simulink model "DCmotor_single_loop"  (R2023a)
settings: Solver=VariableStepAuto  StartTime=0.0  StopTime=3  RelTol=1e-3
libraries: spsIGBTDiodeLib x4, spsDCVoltageSourceLib x2, spsDCMachineLib x1, spsTriangleGeneratorLib x1, spsVoltageMeasurementLib x1, spspowerguiLib x1
settings Model: Creator=搬砖工卢卡斯  LastModifiedBy=LabourerLucas
settings DebuggingCC: UnconnectedInputMsg=warning  UnconnectedOutputMsg=warning  UnconnectedLineMsg=warning
settings ModelReferenceCC: EnableRefExpFcnMdlSchedulingChecks=on
settings RTWCC: DLArmComputeVersion=19.05

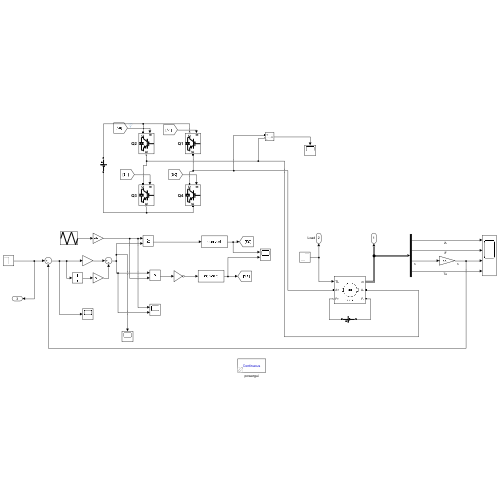
[thumbnail: Simulink's stored preview of the top-level diagram]
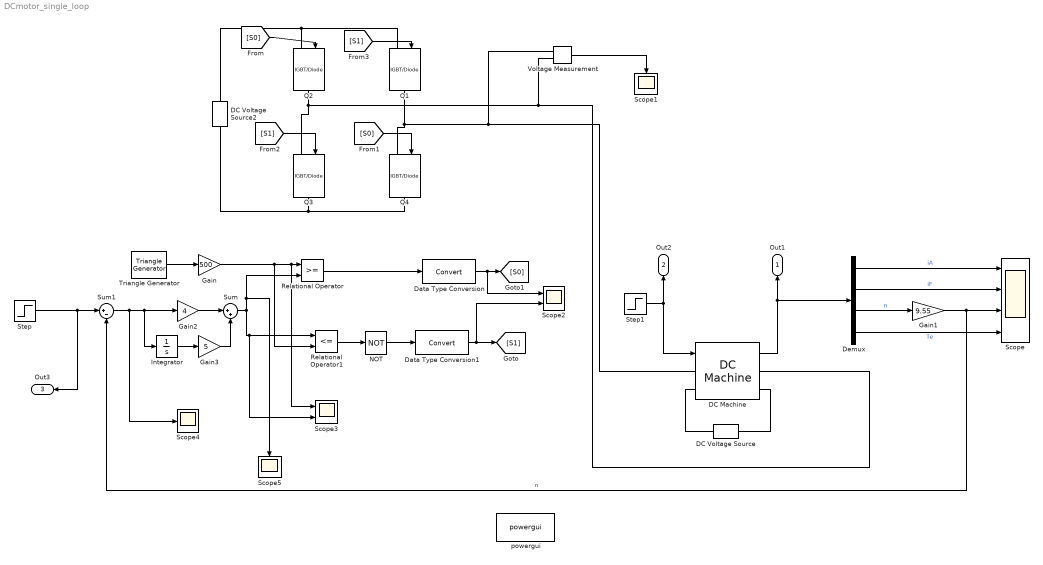
== system DCmotor_single_loop ==
  DC Machine : spsDCMachineLib/DC Machine  PresetModel=No  MechanicalLoad=Torque TL  FieldType=Wound  ShowDetailedParameters=on  MeasurementBus=on  RLa="[ 0.6  0.012]"  RLf="[ 240  120]"  Laf=1.8  MachineConstant=Torque constant (N.m/A)  Ke=1.8  Kt=1.8  J=1  Bm=1  Tf=0  w0=1  Ifinit=0.916666666666667  TsPowergui=0  TsBlock=-1
  DC Voltage Source : spsDCVoltageSourceLib/DC Voltage Source  Amplitude=220  Measurements=None
  DC Voltage Source2 : spsDCVoltageSourceLib/DC Voltage Source  Amplitude=300  Measurements=None
  Data Type Conversion : DataTypeConversion  SaturateOnIntegerOverflow=off  RndMeth=Floor
  Data Type Conversion1 : DataTypeConversion  SaturateOnIntegerOverflow=off  RndMeth=Floor
  Demux : Demux
  Gain : Gain  Gain=500
  Gain1 : Gain  Gain=9.55
  Gain2 : Gain  Gain=4
  Gain3 : Gain  Gain=5
  Integrator : Integrator
  NOT : Logic  Operator=NOT  IconShape=distinctive  AllPortsSameDT=off  OutDataTypeStr=boolean
  Q{1..4} (4 alike) : spsIGBTDiodeLib/IGBT//Diode  Ron=1e-3  Rs=1e5  Cs=inf  Measurements=off
  Relational Operator : RelationalOperator  OutDataTypeStr=boolean  RndMeth=Simplest  InputSameDT=off
  Relational Operator1 : RelationalOperator  Operator=<=  OutDataTypeStr=boolean  RndMeth=Simplest  InputSameDT=off
  Scope : Scope  NumInputPorts=4
  Scope1 : Scope
  Scope2 : Scope  NumInputPorts=2
  Scope3 : Scope  NumInputPorts=2
  Scope4 : Scope
  Scope5 : Scope
  Step : Step  Time=1.5  Before=1200  After=500  SampleTime=0
  Step1 : Step  Time=1.5  After=0  SampleTime=0
  Sum : Sum  Inputs=|++
  Sum1 : Sum  Inputs=|+-
  Triangle Generator : spsTriangleGeneratorLib/Triangle Generator  Freq=1e3  Phase=90  Ts=0
  Voltage Measurement : spsVoltageMeasurementLib/Voltage Measurement  PhasorSimulation=off  OutputType=Complex  PSBequivalent=0
  powergui : spspowerguiLib/powergui  Priority=1  SimulationMode=Continuous  SampleTime=1e-6  frequency=60  Iterations=50  frequencyindice=0  Pbase=100e6  ErrMax=1e-4  UnitsV=kV  UnitsW=MW  buscounter=0  FunctionMessages=off  echomessages=off  EnableUseOfTLC=off  CurrentSourceSwitches=off  DisableSnubberDevices=off  DisableRonSwitches=off  DisableVfSwitches=off  DisplayEquations=off  AutomaticDiscreteSolvers=off  SolverType=Tustin/Backward Euler (TBE)  Interpol=off  ExternalGateDelay=off  methode=off  Ts=100  x0status=blocks  SPID=on  SwTol=0  HookPort=off  NonlinearTolerance=1e-4  nMaxIteration=100  ContinueOnMaxIteration=off  RestoreLinks=warning  ResistiveCurrentMeasurement=off  Frange=[0:2:500]  Ylog=off  Xlog=on  ShowGrid=off  save=off  variable=ZData  structure=0  ZoomFFT=off  StartTime=0.0  cycles=1  DisplayStyle=1  fundamental=60  FreqAxis=off  MaxFrequency=1000  frequencyindicesteady=1  RmsSteady=1  display=off
  Out1 : Outport
  Out2 : Outport  Port=2  SignalName=Load
  Out3 : Outport  Port=3
  wires:
  Step1/1 -> DC Machine/1, Out2/1
  DC Machine/1 -> Out1/1, Demux/1
  Demux/2 -> Scope/2  "iF"
  Demux/4 -> Scope/4  "Te"
  Demux/1 -> Scope/1  "iA"
  Gain1/1 -> Scope/3, Sum1/2  "n"
  Demux/3 -> Gain1/1  "n"
  [S1] -> Q1/1
  Data Type Conversion1/1 -> Scope2/2, [S1]
  Relational Operator1/1 -> NOT/1
  [S0] -> Q4/1
  [S1] -> Q3/1
  NOT/1 -> Data Type Conversion1/1
  [S0] -> Q2/1
  Data Type Conversion/1 -> Scope2/1, [S0]
  Relational Operator/1 -> Data Type Conversion/1
  Triangle Generator/1 -> Gain/1
  Sum1/1 -> Integrator/1, Gain2/1, Scope4/1
  Gain/1 -> Relational Operator1/2, Scope3/1, Relational Operator/1
  Voltage Measurement/1 -> Scope1/1
  Step/1 -> Out3/1, Sum1/1
  Gain2/1 -> Sum/1
  Sum/1 -> Scope5/1, Relational Operator/2, Scope3/2, Relational Operator1/1
  Gain3/1 -> Sum/2
  Integrator/1 -> Gain3/1
  connections:
  DC Voltage Source/RConn1 -- DC Machine/LConn2
  DC Voltage Source/LConn1 -- DC Machine/RConn2
  Q1/LConn1 -- Q2/LConn1 -- DC Voltage Source2/RConn1
  Q4/RConn1 -- Q3/RConn1 -- DC Voltage Source2/LConn1
  Voltage Measurement/LConn1 -- Q1/RConn1 -- Q4/LConn1 -- DC Machine/LConn1
  Q2/RConn1 -- Q3/LConn1 -- Voltage Measurement/LConn2 -- DC Machine/RConn1
